simulink model "Lab1"  (R2020b)
settings: Solver=VariableStepAuto  StartTime=0.0  StopTime=0.35  RelTol=1e-3
model workspace (MAT data in the model file):
  J = 3.2284e-06
  K = 0.0274
  Kd = 0.0022
  Ki = 5.4
  Kp = 0.5
  L = 2.75e-06
  R = 4
  Sig = Simulink.Signal
  Sig.DataType = 'auto'
  Sig.Dimensions = -1
  Sig.DimensionsMode = 'auto'
  Sig.Complexity = 'auto'
  Sig.SampleTime = -1
  Sig.SamplingMode = 'auto'
  b = 3.5077e-06
settings Model: Creator=kevin  LastModifiedBy=kevin

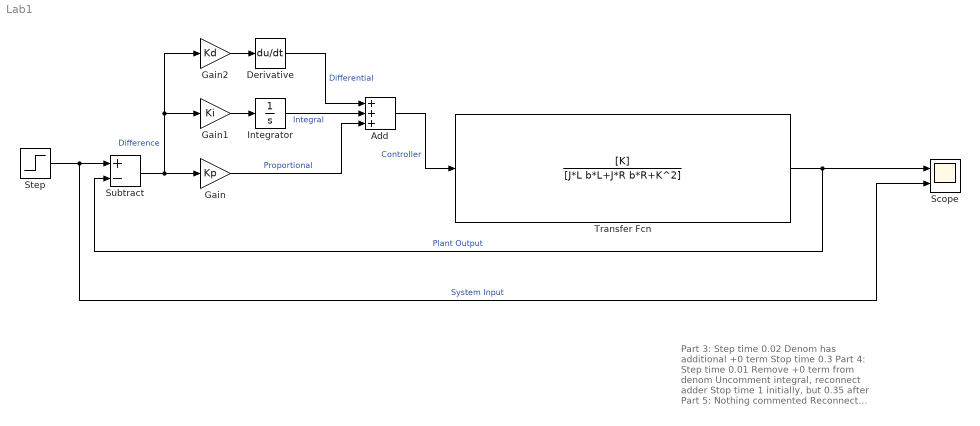
== system Lab1 ==
  note: Part 3:
      | Step time 0.02
      | Denom has additional +0 term
      | Stop time 0.3
      |
      | Part 4:
      | Step time 0.01
      | Remove +0 term from denom
      | Uncomment integral, reconnect adder
      | Stop time 1 initially, but 0.35 after
      |
      | Part 5:
      | Nothing commented
      | Reconnect everything
      | Zoom into noise
      | Stop time 0.35s
  Add : Sum  Inputs=+++
  Derivative : Derivative
  Gain : Gain  Gain=Kp
  Gain1 : Gain  Gain=Ki
  Gain2 : Gain  Gain=Kd
  Integrator : Integrator
  Scope : Scope  NumInputPorts=2
  Step : Step  Time=0.01  After=60  SampleTime=0
  Subtract : Sum  Inputs=+-
  Transfer Fcn : TransferFcn  Numerator=[K]  Denominator=[J*L b*L+J*R b*R+K^2]
  wires:
  Step/1 -> Subtract/1, Scope/2  "System Input"
  Transfer Fcn/1 -> Subtract/2, Scope/1  "Plant Output"
  Subtract/1 -> Gain2/1, Gain1/1, Gain/1  "Difference"
  Gain/1 -> Add/3  "Proportional"
  Gain1/1 -> Integrator/1
  Integrator/1 -> Add/2  "Integral"
  Add/1 -> Transfer Fcn/1  "Controller"
  Gain2/1 -> Derivative/1
  Derivative/1 -> Add/1  "Differential"
